simulink library "lib_Gimbal"  (R2017a)
settings: Solver=VariableStepAuto  StartTime=0.0  StopTime=10.0  RelTol=1e-3
undefined symbols (not defined in the file or in its folder): HIL_Data, HIL_Sample_Time, National_Instruments, PCIe, Standard_Devices, UDP_Protocol
libraries: sldrtlib x6, lib_Gimbal x5, sharedtransform x1
settings Model: Creator=m.hiepp  LastModifiedBy=m.hiepp
settings SFSimCC: SimUseLocalCustomCode=on
settings RTWCC: RTWUseLocalCustomCode=on

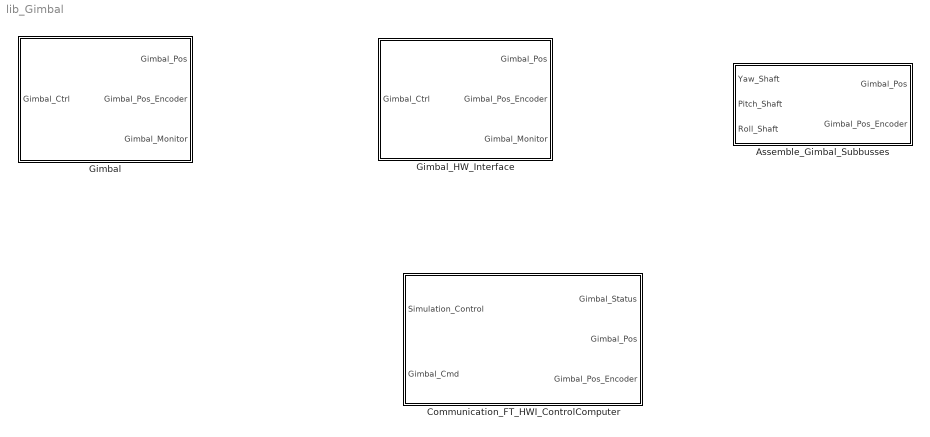
== system lib_Gimbal ==
  Assemble_Gimbal_Subbusses : Subsystem
  Communication_FT_HWI_ControlComputer : Subsystem  mask{FTHWICC=HIL_Data.Gimbal.FTHWICC}
      mask prompts: FTHWICC "FT HWI CC Connection Data"
  Gimbal : Subsystem  Variant=on
  Gimbal_HW_Interface : Subsystem  mask{HW=HIL_Data.Gimbal.HW}
      mask prompts: HW "HW Data"

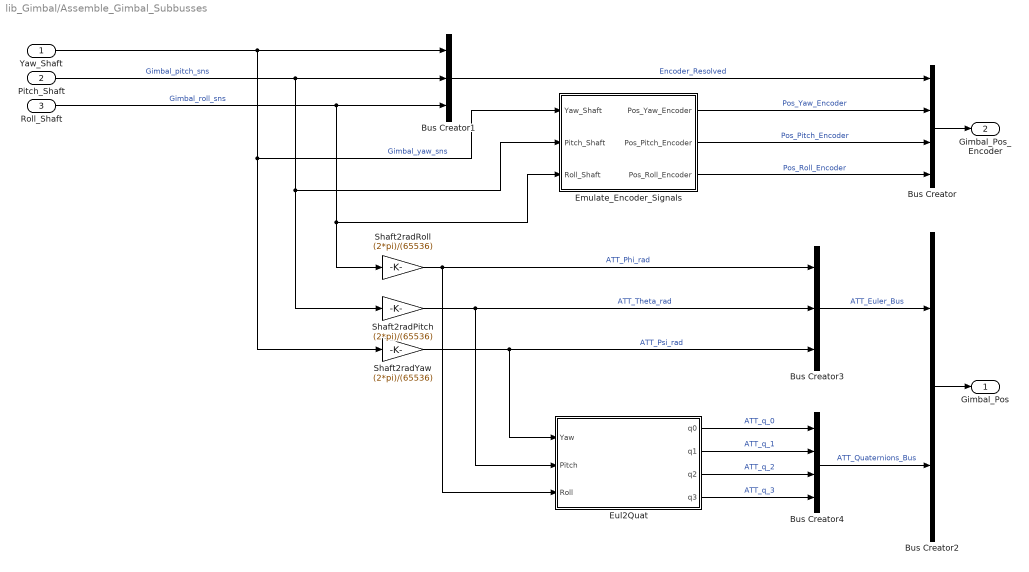
== system lib_Gimbal/Assemble_Gimbal_Subbusses ==
  Yaw_Shaft : Inport
  Pitch_Shaft : Inport  Port=2
  Roll_Shaft : Inport  Port=3
  Bus Creator : BusCreator  Inputs=4  OutDataTypeStr=Bus: Gimbal_Encoder_Bus
  Bus Creator1 : BusCreator  Inputs=3  OutDataTypeStr=Bus: Encoder_Resolved_Bus
  Bus Creator2 : BusCreator  Inputs=2  OutDataTypeStr=Bus: Attitude_States_Bus
  Bus Creator3 : BusCreator  Inputs=3  OutDataTypeStr=Bus: ATT_Euler_Bus
  Bus Creator4 : BusCreator  Inputs=4  OutDataTypeStr=Bus: ATT_Quaternions_Bus
  Emulate_Encoder_Signals : Subsystem
  Eul2Quat : Subsystem
  Shaft2radPitch : Gain  Gain=(2*pi)/(65536)
  Shaft2radRoll : Gain  Gain=(2*pi)/(65536)
  Shaft2radYaw : Gain  Gain=(2*pi)/(65536)
  Gimbal_Pos : Outport  OutDataTypeStr=Bus: Gimbal_Attitude_Bus
  Gimbal_Pos_Encoder : Outport  Port=2  OutDataTypeStr=Bus: Gimbal_Encoder_Bus
  wires:
  Roll_Shaft/1 -> Emulate_Encoder_Signals/3(Roll_Shaft), Shaft2radRoll/1, Bus Creator1/3  "Gimbal_roll_sns"
  Yaw_Shaft/1 -> Emulate_Encoder_Signals/1(Yaw_Shaft), Shaft2radYaw/1, Bus Creator1/1  "Gimbal_yaw_sns"
  Shaft2radPitch/1 -> Eul2Quat/2(Pitch), Bus Creator3/2  "ATT_Theta_rad"
  Bus Creator2/1 -> Gimbal_Pos/1
  Eul2Quat/4(q3) -> Bus Creator4/4  "ATT_q_3"
  Bus Creator/1 -> Gimbal_Pos_Encoder/1
  Eul2Quat/1(q0) -> Bus Creator4/1  "ATT_q_0"
  Pitch_Shaft/1 -> Emulate_Encoder_Signals/2(Pitch_Shaft), Shaft2radPitch/1, Bus Creator1/2  "Gimbal_pitch_sns"
  Eul2Quat/2(q1) -> Bus Creator4/2  "ATT_q_1"
  Bus Creator3/1 -> Bus Creator2/1  "ATT_Euler_Bus"
  Bus Creator4/1 -> Bus Creator2/2  "ATT_Quaternions_Bus"
  Bus Creator1/1 -> Bus Creator/1  "Encoder_Resolved"
  Shaft2radRoll/1 -> Eul2Quat/3(Roll), Bus Creator3/1  "ATT_Phi_rad"
  Shaft2radYaw/1 -> Eul2Quat/1(Yaw), Bus Creator3/3  "ATT_Psi_rad"
  Eul2Quat/3(q2) -> Bus Creator4/3  "ATT_q_2"
  Emulate_Encoder_Signals/1(Pos_Yaw_Encoder) -> Bus Creator/2  "Pos_Yaw_Encoder"
  Emulate_Encoder_Signals/2(Pos_Pitch_Encoder) -> Bus Creator/3  "Pos_Pitch_Encoder"
  Emulate_Encoder_Signals/3(Pos_Roll_Encoder) -> Bus Creator/4  "Pos_Roll_Encoder"

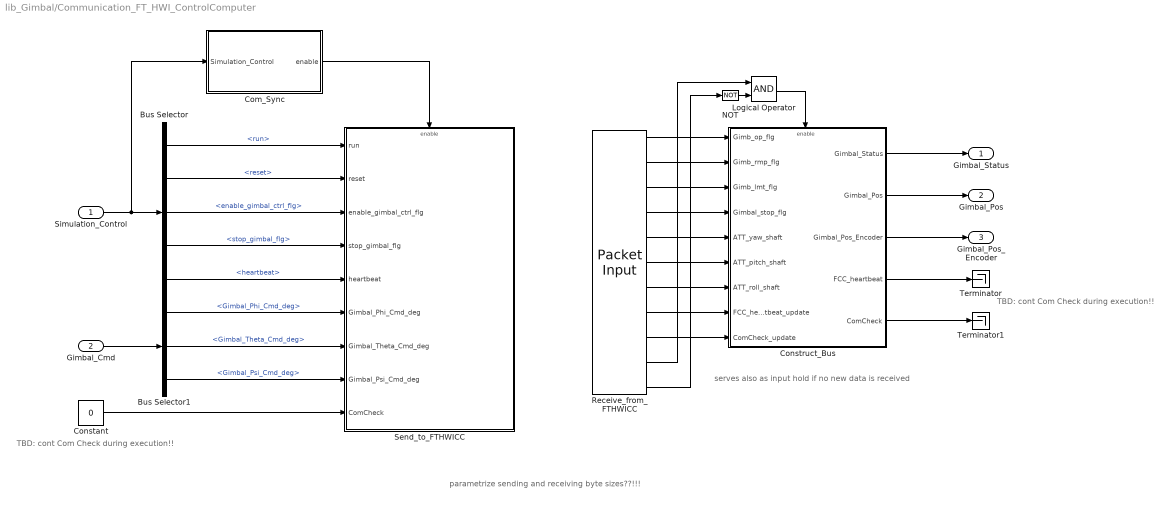
== system lib_Gimbal/Communication_FT_HWI_ControlComputer ==
  note: parametrize sending and receiving byte sizes??!!!
  note: TBD: cont Com Check during execution!!
  note: serves also as input hold if no new data is received
  note: TBD: cont Com Check during execution!!
  Simulation_Control : Inport  OutDataTypeStr=Bus: Simulation_Ctrl_Bus
  Gimbal_Cmd : Inport  Port=2  OutDataTypeStr=Bus: Gimbal_Cmd_Bus
  Bus Selector : BusSelector  OutputSignals=run,reset,HW_Ctrl.enable_gimbal_ctrl_flg,HW_Ctrl.stop_gimbal_flg,heartbeat
  Bus Selector1 : BusSelector  OutputSignals=Gimbal_Phi_Cmd_deg,Gimbal_Theta_Cmd_deg,Gimbal_Psi_Cmd_deg
  Com_Sync : Subsystem
  Constant : Constant  Value=0
  Construct_Bus : Subsystem
  Logical Operator : Logic  AllPortsSameDT=off  OutDataTypeStr=boolean
  NOT : Logic  Operator=NOT  IconShape=distinctive  AllPortsSameDT=off  OutDataTypeStr=boolean
  Receive_from_FTHWICC : sldrtlib/Packet Input  SampleTime=FTHWICC.SampTime  MaxMissedTicks=FTHWICC.MaxMissedTicks  ShowMissedTicks=off  YieldWhenWaiting=on  DrvName=Standard_Devices/UDP_Protocol  DrvAddress=36880  DrvOptions=[0 36864 0 0 0 0 0 0 0 0 0 0 0 0 0 0 0 0 0 0 0 0 0 0 0 0 0 0 0 0 0 0 0 0 0 0 0 0 0 0 0 0 0 0 0 0 0 0 0 0 0 0 0 0 0 0 0 0 0 0 0 0 0 0 0 0 0 0 0 0 0 0 0 0 0 0 0 0 0 0 0 0 0 0 0 0 0 0 0 0 0 0 0 0 0 0 0 0 0 0 0 0 0 0 0 0 0 0 0 0 0 0 0 0 0 0 0 0 0 0 0 0 0 0 0 0 0 0 0 0 0 0 0 0 0 0 0 0 0 0 0 0 0 0 0 0 0 0 0 0 0 0 0 0 0 0 0 0 0 0 0 0 0 0 0 0 0 0 0 0 0 0 0 0 0 0 0 0 0 0 0 0 0 0 0 0 0 0 0 0 0 0 0 0 0 0 0 0 0 0 0 0 0 0 0 0 0 0 0 0 0 0 0 0 0 0 0 0 0 0 0 0 0 0 0 0 0 0 0 0 0 0 0 0 0 0 0 0 0 0 0 0 0 0 0 0 0 0 0 0 0 0 0 0 0 0]  PacketSize=66  DataTypes={'double','double','double','double','double','double','double','uint16','double'}  ShowReady=on  ShowError=on  PacketID=1  ByteOrder=1  ShowTimestamp=off
      settings: AttributesFormatString=UDP Protocol [36880]  SourceProductName=Simulink Desktop Real-Time
  Send_to_FTHWICC : Subsystem
  Terminator : Terminator
  Terminator1 : Terminator
  Gimbal_Status : Outport  OutDataTypeStr=Bus: Gimbal_Status_Bus
  Gimbal_Pos : Outport  Port=2  OutDataTypeStr=Bus: Gimbal_Attitude_Bus
  Gimbal_Pos_Encoder : Outport  Port=3  OutDataTypeStr=Bus: Gimbal_Encoder_Bus
  wires:
  Simulation_Control/1 -> Com_Sync/1(Simulation_Control), Bus Selector/1
  Gimbal_Cmd/1 -> Bus Selector1/1
  Receive_from_FTHWICC/1 -> Construct_Bus/1(Gimb_op_flg)
  Receive_from_FTHWICC/2 -> Construct_Bus/2(Gimb_rmp_flg)
  Receive_from_FTHWICC/3 -> Construct_Bus/3(Gimb_lmt_flg)
  Receive_from_FTHWICC/4 -> Construct_Bus/4(Gimbal_stop_flg)
  Receive_from_FTHWICC/5 -> Construct_Bus/5(ATT_yaw_shaft)
  Receive_from_FTHWICC/6 -> Construct_Bus/6(ATT_pitch_shaft)
  Receive_from_FTHWICC/7 -> Construct_Bus/7(ATT_roll_shaft)
  Construct_Bus/1(Gimbal_Status) -> Gimbal_Status/1
  Construct_Bus/2(Gimbal_Pos) -> Gimbal_Pos/1
  Construct_Bus/3(Gimbal_Pos_Encoder) -> Gimbal_Pos_Encoder/1
  NOT/1 -> Logical Operator/2
  Receive_from_FTHWICC/10 -> Logical Operator/1
  Receive_from_FTHWICC/11 -> NOT/1
  Logical Operator/1 -> Construct_Bus/Enable
  Bus Selector/1 -> Send_to_FTHWICC/1(run)  "<run>"
  Bus Selector/2 -> Send_to_FTHWICC/2(reset)  "<reset>"
  Bus Selector/3 -> Send_to_FTHWICC/3(enable_gimbal_ctrl_flg)  "<enable_gimbal_ctrl_flg>"
  Bus Selector/4 -> Send_to_FTHWICC/4(stop_gimbal_flg)  "<stop_gimbal_flg>"
  Bus Selector/5 -> Send_to_FTHWICC/5(heartbeat)  "<heartbeat>"
  Bus Selector1/1 -> Send_to_FTHWICC/6(Gimbal_Phi_Cmd_deg)  "<Gimbal_Phi_Cmd_deg>"
  Bus Selector1/2 -> Send_to_FTHWICC/7(Gimbal_Theta_Cmd_deg)  "<Gimbal_Theta_Cmd_deg>"
  Bus Selector1/3 -> Send_to_FTHWICC/8(Gimbal_Psi_Cmd_deg)  "<Gimbal_Psi_Cmd_deg>"
  Com_Sync/1(enable) -> Send_to_FTHWICC/Enable
  Constant/1 -> Send_to_FTHWICC/9(ComCheck)
  Receive_from_FTHWICC/8 -> Construct_Bus/8(FCC_heartbeat_update)
  Receive_from_FTHWICC/9 -> Construct_Bus/9(ComCheck_update)
  Construct_Bus/4(FCC_heartbeat) -> Terminator/1
  Construct_Bus/5(ComCheck) -> Terminator1/1

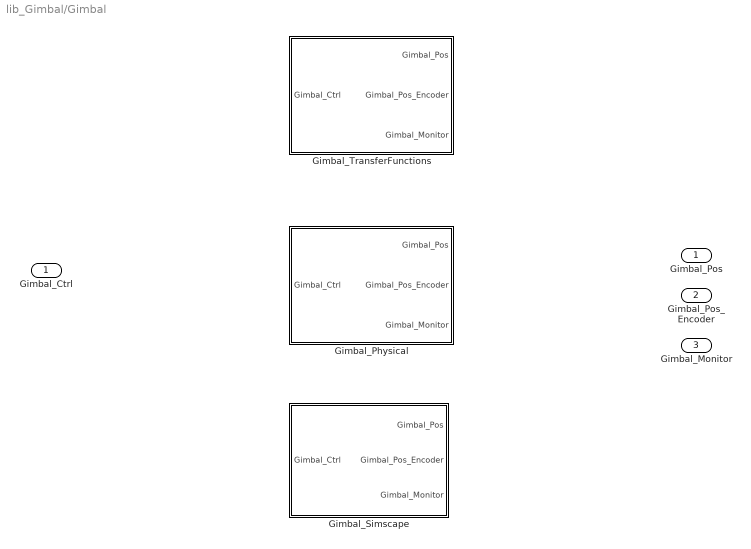
== system lib_Gimbal/Gimbal ==
  Gimbal_Ctrl : Inport  OutDataTypeStr=Bus: Gimbal_Ctrl_Bus
  Gimbal_Physical : Subsystem  VariantControl=VSS_GIMBAL_PH
  Gimbal_Simscape : Subsystem  VariantControl=VSS_GIMBAL_SC
  Gimbal_TransferFunctions : Subsystem  VariantControl=VSS_GIMBAL_TF  mask{TF=HIL_Data.Gimbal.TF}
      mask prompts: TF "Transfer_Functions"
  Gimbal_Pos : Outport  OutDataTypeStr=Bus: Gimbal_Attitude_Bus
  Gimbal_Pos_Encoder : Outport  Port=2  OutDataTypeStr=Bus: Gimbal_Encoder_Bus
  Gimbal_Monitor : Outport  Port=3  OutDataTypeStr=Bus: Gimbal_Monitor_Bus

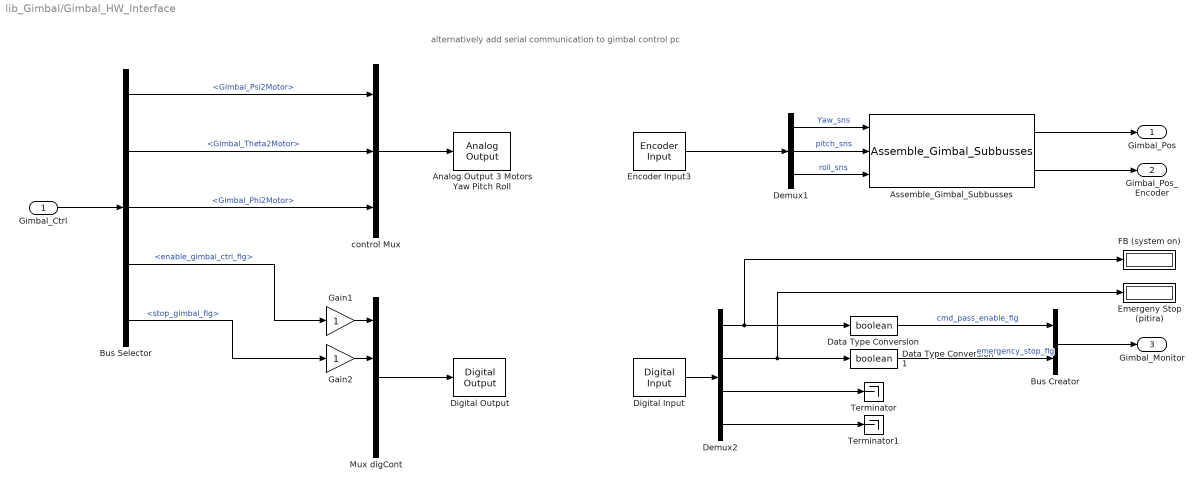
== system lib_Gimbal/Gimbal_HW_Interface ==
  note: alternatively add serial communication to gimbal control pc
  Gimbal_Ctrl : Inport  OutDataTypeStr=Bus: Gimbal_Ctrl_Bus
  Analog Output 3 Motors Yaw Pitch Roll : sldrtlib/Analog Output  SampleTime=HW.SampTime  MaxMissedTicks=HW.MaxMissTick  ShowMissedTicks=off  YieldWhenWaiting=off  DrvName=National_Instruments/PCIe-6353  DrvAddress=4294967295  DrvOptions=[0 15 0 2 2 2 2]  Channels=[1:3]  RangeMode=1  VoltRange=1  InitialValue=0  FinalValue=0
      settings: AttributesFormatString=National Instruments\nPCIe-6353 [auto]  SourceProductName=Simulink Desktop Real-Time
  Assemble_Gimbal_Subbusses : lib_Gimbal/Assemble_Gimbal_Subbusses  SystemSampleTime=-1
  Bus Creator : BusCreator  Inputs=2  OutDataTypeStr=Bus: Gimbal_Monitor_Bus
  Bus Selector : BusSelector  OutputSignals=Gimbal_Psi2Motor,Gimbal_Theta2Motor,Gimbal_Phi2Motor,enable_gimbal_ctrl_flg,stop_gimbal_flg
  Data Type Conversion : DataTypeConversion  OutDataTypeStr=boolean
  Data Type Conversion1 : DataTypeConversion  OutDataTypeStr=boolean
  Demux1 : Demux  Outputs=3
  Demux2 : Demux
  Digital Input : sldrtlib/Digital Input  SampleTime=HW.SampTime  MaxMissedTicks=HW.MaxMissTick  ShowMissedTicks=off  YieldWhenWaiting=off  DrvName=National_Instruments/PCIe-6353  DrvAddress=4294967295  DrvOptions=[0 15 0 2 2 2 2]  Channels=[5:8]  BitMode=1  DataType=1
      settings: AttributesFormatString=National Instruments\nPCIe-6353 [auto]  SourceProductName=Simulink Desktop Real-Time  SourceProductBaseCode=WT
  Digital Output : sldrtlib/Digital Output  SampleTime=HW.SampTime  MaxMissedTicks=HW.MaxMissTick  ShowMissedTicks=off  YieldWhenWaiting=off  DrvName=National_Instruments/PCIe-6353  DrvAddress=4294967295  DrvOptions=[0 15 0 2 2 2 2]  Channels=[1:4]  BitMode=1  InitialValue=[]  FinalValue=[]
      settings: AttributesFormatString=National Instruments\nPCIe-6353 [auto]  SourceProductName=Simulink Desktop Real-Time  SourceProductBaseCode=WT
  Emergeny Stop (pitira) : Display
      settings: Tag=SampTime
  Encoder Input3 : sldrtlib/Encoder Input  SampleTime=HW.SampTime  MaxMissedTicks=HW.MaxMissTick  ShowMissedTicks=off  YieldWhenWaiting=off  DrvName=National_Instruments/PCIe-6353  DrvAddress=4294967295  DrvOptions=[0 15 0 2 2 2 2]  Channels=[1:3]  QuadMode=3  IndexPulse=1  InputFilter=Inf  DataType=1
      settings: AttributesFormatString=National Instruments\nPCIe-6353 [auto]  SourceProductName=Simulink Desktop Real-Time
  FB (system on) : Display
      settings: Tag=SampTime
  Gain1 : Gain
  Gain2 : Gain
  Mux digCont : Mux
  Terminator : Terminator
  Terminator1 : Terminator
  control Mux : Mux  Inputs=3
  Gimbal_Pos : Outport  OutDataTypeStr=Bus: Gimbal_Attitude_Bus
  Gimbal_Pos_Encoder : Outport  Port=2  OutDataTypeStr=Bus: Gimbal_Encoder_Bus
  Gimbal_Monitor : Outport  Port=3  OutDataTypeStr=Bus: Gimbal_Monitor_Bus
  wires:
  Assemble_Gimbal_Subbusses/2 -> Gimbal_Pos_Encoder/1
  Gimbal_Ctrl/1 -> Bus Selector/1
  Assemble_Gimbal_Subbusses/1 -> Gimbal_Pos/1
  control Mux/1 -> Analog Output 3 Motors Yaw Pitch Roll/1
  Demux1/3 -> Assemble_Gimbal_Subbusses/3  "roll_sns"
  Demux1/1 -> Assemble_Gimbal_Subbusses/1  "Yaw_sns"
  Demux1/2 -> Assemble_Gimbal_Subbusses/2  "pitch_sns"
  Encoder Input3/1 -> Demux1/1
  Bus Selector/1 -> control Mux/1  "<Gimbal_Psi2Motor>"
  Bus Selector/2 -> control Mux/2  "<Gimbal_Theta2Motor>"
  Bus Selector/3 -> control Mux/3  "<Gimbal_Phi2Motor>"
  Demux2/1 -> Data Type Conversion/1, FB (system on)/1
  Digital Input/1 -> Demux2/1
  Mux digCont/1 -> Digital Output/1
  Demux2/2 -> Data Type Conversion1/1, Emergeny Stop (pitira)/1
  Bus Creator/1 -> Gimbal_Monitor/1
  Data Type Conversion/1 -> Bus Creator/1  "cmd_pass_enable_flg"
  Data Type Conversion1/1 -> Bus Creator/2  "emergency_stop_flg"
  Demux2/3 -> Terminator/1
  Demux2/4 -> Terminator1/1
  Bus Selector/4 -> Gain1/1  "<enable_gimbal_ctrl_flg>"
  Gain1/1 -> Mux digCont/1
  Gain2/1 -> Mux digCont/2
  Bus Selector/5 -> Gain2/1  "<stop_gimbal_flg>"

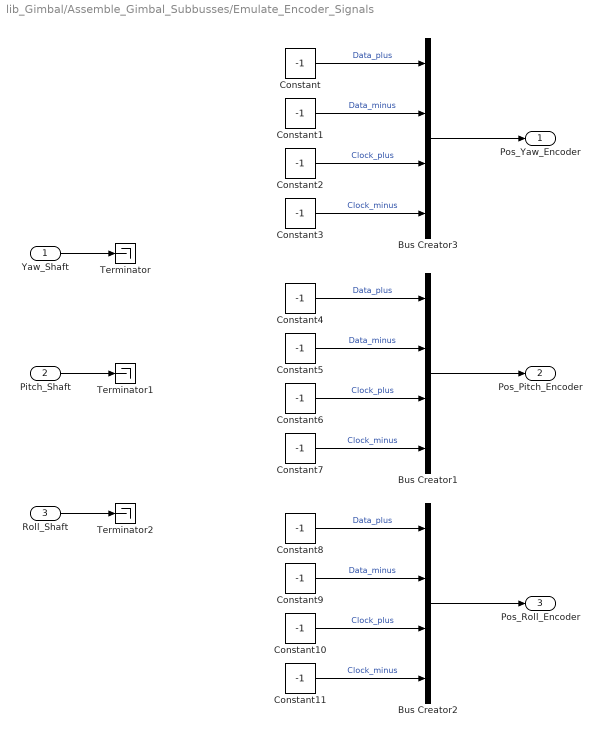
== system lib_Gimbal/Assemble_Gimbal_Subbusses/Emulate_Encoder_Signals ==
  Yaw_Shaft : Inport
  Pitch_Shaft : Inport  Port=2
  Roll_Shaft : Inport  Port=3
  Bus Creator1 : BusCreator  Inputs=4  OutDataTypeStr=Bus: Encoder_Signal_Bus
  Bus Creator2 : BusCreator  Inputs=4  OutDataTypeStr=Bus: Encoder_Signal_Bus
  Bus Creator3 : BusCreator  Inputs=4  OutDataTypeStr=Bus: Encoder_Signal_Bus
  Constant{,1..11} (12 alike) : Constant  Value=-1
  Terminator : Terminator
  Terminator1 : Terminator
  Terminator2 : Terminator
  Pos_Yaw_Encoder : Outport  OutDataTypeStr=Bus: Encoder_Signal_Bus
  Pos_Pitch_Encoder : Outport  Port=2  OutDataTypeStr=Bus: Encoder_Signal_Bus
  Pos_Roll_Encoder : Outport  Port=3  OutDataTypeStr=Bus: Encoder_Signal_Bus
  wires:
  Bus Creator2/1 -> Pos_Roll_Encoder/1
  Yaw_Shaft/1 -> Terminator/1
  Pitch_Shaft/1 -> Terminator1/1
  Roll_Shaft/1 -> Terminator2/1
  Bus Creator3/1 -> Pos_Yaw_Encoder/1
  Bus Creator1/1 -> Pos_Pitch_Encoder/1
  Constant/1 -> Bus Creator3/1  "Data_plus"
  Constant11/1 -> Bus Creator2/4  "Clock_minus"
  Constant10/1 -> Bus Creator2/3  "Clock_plus"
  Constant9/1 -> Bus Creator2/2  "Data_minus"
  Constant8/1 -> Bus Creator2/1  "Data_plus"
  Constant7/1 -> Bus Creator1/4  "Clock_minus"
  Constant6/1 -> Bus Creator1/3  "Clock_plus"
  Constant5/1 -> Bus Creator1/2  "Data_minus"
  Constant3/1 -> Bus Creator3/4  "Clock_minus"
  Constant4/1 -> Bus Creator1/1  "Data_plus"
  Constant2/1 -> Bus Creator3/3  "Clock_plus"
  Constant1/1 -> Bus Creator3/2  "Data_minus"

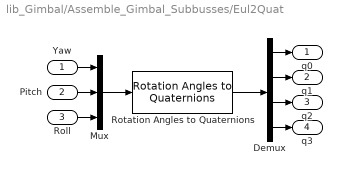
== system lib_Gimbal/Assemble_Gimbal_Subbusses/Eul2Quat ==
  Yaw : Inport
  Pitch : Inport  Port=2
  Roll : Inport  Port=3
  Demux : Demux
  Mux : Mux  Inputs=3
  Rotation Angles to Quaternions : sharedtransform/Rotation Angles to Quaternions  rotationOrder=XYZ
      settings: SourceProductName=Aerospace Blockset  SourceProductBaseCode=AE
  q0 : Outport
  q1 : Outport  Port=2
  q2 : Outport  Port=3
  q3 : Outport  Port=4
  wires:
  Demux/2 -> q1/1
  Pitch/1 -> Mux/2
  Rotation Angles to Quaternions/1 -> Demux/1
  Mux/1 -> Rotation Angles to Quaternions/1
  Demux/4 -> q3/1
  Roll/1 -> Mux/3
  Demux/3 -> q2/1
  Yaw/1 -> Mux/1
  Demux/1 -> q0/1

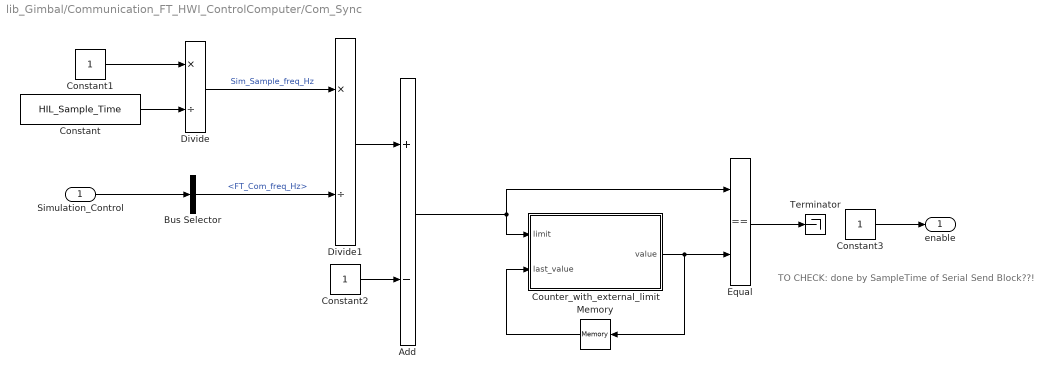
== system lib_Gimbal/Communication_FT_HWI_ControlComputer/Com_Sync ==
  note: TO CHECK: done by SampleTime of Serial Send Block??!
  Simulation_Control : Inport  OutDataTypeStr=Bus: Simulation_Ctrl_Bus
  Add : Sum  Inputs=+-
  Bus Selector : BusSelector  OutputSignals=COM_Ctrl.FT_Com_freq_Hz
  Constant : Constant  Value=HIL_Sample_Time
  Constant1 : Constant
  Constant2 : Constant
  Constant3 : Constant  OutDataTypeStr=boolean
  Counter_with_external_limit : MATLAB Function  TreatAsAtomicUnit=on
  Divide : Product  Inputs=*/
  Divide1 : Product  Inputs=*/
  Equal : RelationalOperator  Operator===  OutDataTypeStr=boolean  RndMeth=Simplest
  Memory : Memory  X0=-1
  Terminator : Terminator
  enable : Outport
  wires:
  Simulation_Control/1 -> Bus Selector/1
  Constant/1 -> Divide/2
  Constant1/1 -> Divide/1
  Divide/1 -> Divide1/1  "Sim_Sample_freq_Hz"
  Bus Selector/1 -> Divide1/2  "<FT_Com_freq_Hz>"
  Divide1/1 -> Add/1
  Constant2/1 -> Add/2
  Counter_with_external_limit/1(value) -> Memory/1, Equal/2
  Memory/1 -> Counter_with_external_limit/2(last_value)
  Add/1 -> Equal/1, Counter_with_external_limit/1(limit)
  Equal/1 -> Terminator/1
  Constant3/1 -> enable/1

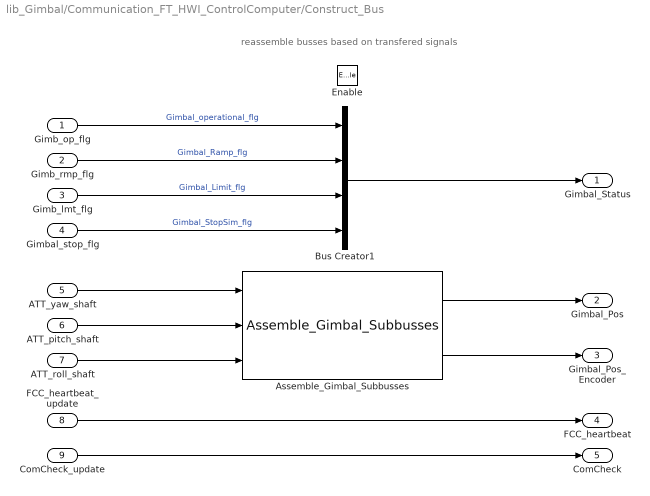
== system lib_Gimbal/Communication_FT_HWI_ControlComputer/Construct_Bus ==
  note: reassemble busses based on transfered signals
  Gimb_op_flg : Inport
  Gimb_rmp_flg : Inport  Port=2
  Gimb_lmt_flg : Inport  Port=3
  Gimbal_stop_flg : Inport  Port=4
  ATT_yaw_shaft : Inport  Port=5
  ATT_pitch_shaft : Inport  Port=6
  ATT_roll_shaft : Inport  Port=7
  FCC_heartbeat_update : Inport  Port=8
  ComCheck_update : Inport  Port=9
  Enable : EnablePort
  Assemble_Gimbal_Subbusses : lib_Gimbal/Assemble_Gimbal_Subbusses  SystemSampleTime=-1
  Bus Creator1 : BusCreator  Inputs=4
  Gimbal_Status : Outport  OutDataTypeStr=Bus: Gimbal_Status_Bus
  Gimbal_Pos : Outport  Port=2  OutDataTypeStr=Bus: Gimbal_Attitude_Bus
  Gimbal_Pos_Encoder : Outport  Port=3  OutDataTypeStr=Bus: Gimbal_Encoder_Bus
  FCC_heartbeat : Outport  Port=4
  ComCheck : Outport  Port=5
  wires:
  Gimb_lmt_flg/1 -> Bus Creator1/3  "Gimbal_Limit_flg"
  Gimbal_stop_flg/1 -> Bus Creator1/4  "Gimbal_StopSim_flg"
  Gimb_rmp_flg/1 -> Bus Creator1/2  "Gimbal_Ramp_flg"
  Gimb_op_flg/1 -> Bus Creator1/1  "Gimbal_operational_flg"
  Bus Creator1/1 -> Gimbal_Status/1
  ATT_yaw_shaft/1 -> Assemble_Gimbal_Subbusses/1
  ATT_pitch_shaft/1 -> Assemble_Gimbal_Subbusses/2
  ATT_roll_shaft/1 -> Assemble_Gimbal_Subbusses/3
  Assemble_Gimbal_Subbusses/1 -> Gimbal_Pos/1
  Assemble_Gimbal_Subbusses/2 -> Gimbal_Pos_Encoder/1
  FCC_heartbeat_update/1 -> FCC_heartbeat/1
  ComCheck_update/1 -> ComCheck/1

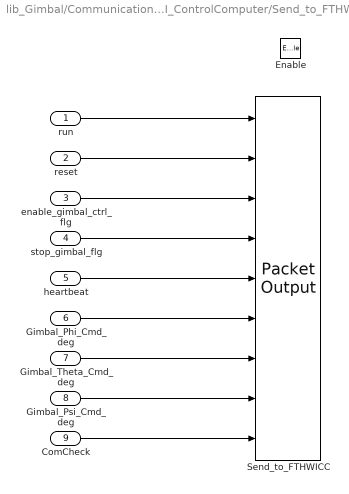
== system lib_Gimbal/Communication_FT_HWI_ControlComputer/Send_to_FTHWICC ==
  run : Inport
  reset : Inport  Port=2
  enable_gimbal_ctrl_flg : Inport  Port=3
  stop_gimbal_flg : Inport  Port=4
  heartbeat : Inport  Port=5
  Gimbal_Phi_Cmd_deg : Inport  Port=6
  Gimbal_Theta_Cmd_deg : Inport  Port=7
  Gimbal_Psi_Cmd_deg : Inport  Port=8
  ComCheck : Inport  Port=9
  Enable : EnablePort
  Send_to_FTHWICC : sldrtlib/Packet Output  SampleTime=1/HIL_Data.Simulation_Ctrl.Com.FT.Com_freq_Hz  MaxMissedTicks=FTHWICC.MaxMissTick  ShowMissedTicks=off  YieldWhenWaiting=on  DrvName=Standard_Devices/UDP_Protocol  DrvAddress=36864  DrvOptions=[0 36880 49 57 50 46 49 54 56 46 49 46 49 53 54 0 0 0 0 0 0 0 0 0 0 0 0 0 0 0 0 0 0 0 0 0 0 0 0 0 0 0 0 0 0 0 0 0 0 0 0 0 0 0 0 0 0 0 0 0 0 0 0 0 0 0 0 0 0 0 0 0 0 0 0 0 0 0 0 0 0 0 0 0 0 0 0 0 0 0 0 0 0 0 0 0 0 0 0 0 0 0 0 0 0 0 0 0 0 0 0 0 0 0 0 0 0 0 0 0 0 0 0 0 0 0 0 0 0 0 0 0 0 0 0 0 0 0 0 0 0 0 0 0 0 0 0 0 0 0 0 0 0 0 0 0 0 0 0 0 0 0 0 0 0 0 0 0 0 0 0 0 0 0 0 0 0 0 0 0 0 0 0 0 0 0 0 0 0 0 0 0 0 0 0 0 0 0 0 0 0 0 0 0 0 0 0 0 0 0 0 0 0 0 0 0 0 0 0 0 0 0 0 0 0 0 0 0 0 0 0 0 0 0 0 0 0 0 0 0 0 0 0 0 0 0 0 0 0 0 0 0 0 0 0 0]  PacketSize=52  DataTypes={'boolean','boolean','double','double','uint16','double','double','double','double'}  ShowReady=off  ShowError=off  PacketID=1  ByteOrder=1  InitialValue=[]  FinalValue=[]
      settings: AttributesFormatString=UDP Protocol [36864]  SourceProductName=Simulink Desktop Real-Time
  wires:
  Gimbal_Psi_Cmd_deg/1 -> Send_to_FTHWICC/8
  heartbeat/1 -> Send_to_FTHWICC/5
  Gimbal_Theta_Cmd_deg/1 -> Send_to_FTHWICC/7
  reset/1 -> Send_to_FTHWICC/2
  Gimbal_Phi_Cmd_deg/1 -> Send_to_FTHWICC/6
  stop_gimbal_flg/1 -> Send_to_FTHWICC/4
  run/1 -> Send_to_FTHWICC/1
  enable_gimbal_ctrl_flg/1 -> Send_to_FTHWICC/3
  ComCheck/1 -> Send_to_FTHWICC/9

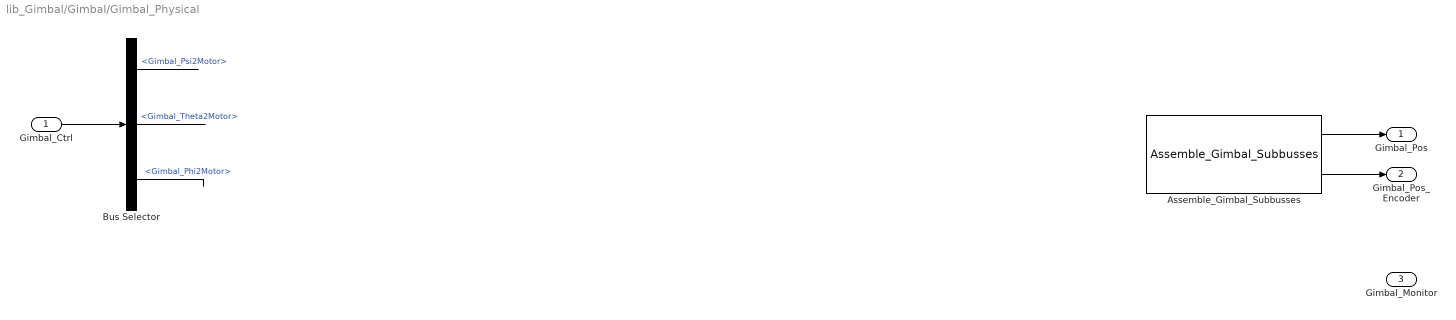
== system lib_Gimbal/Gimbal/Gimbal_Physical ==
  Gimbal_Ctrl : Inport  OutDataTypeStr=Bus: Gimbal_Ctrl_Bus
  Assemble_Gimbal_Subbusses : lib_Gimbal/Assemble_Gimbal_Subbusses  SystemSampleTime=-1
  Bus Selector : BusSelector  OutputSignals=Gimbal_Psi2Motor,Gimbal_Theta2Motor,Gimbal_Phi2Motor
  Gimbal_Pos : Outport  OutDataTypeStr=Bus: Gimbal_Attitude_Bus
  Gimbal_Pos_Encoder : Outport  Port=2  OutDataTypeStr=Bus: Gimbal_Encoder_Bus
  Gimbal_Monitor : Outport  Port=3  OutDataTypeStr=Bus: Gimbal_Monitor_Bus
  wires:
  Gimbal_Ctrl/1 -> Bus Selector/1
  Assemble_Gimbal_Subbusses/1 -> Gimbal_Pos/1
  Assemble_Gimbal_Subbusses/2 -> Gimbal_Pos_Encoder/1
  Bus Selector/1 -> ?  "<Gimbal_Psi2Motor>"
  Bus Selector/2 -> ?  "<Gimbal_Theta2Motor>"
  Bus Selector/3 -> ?  "<Gimbal_Phi2Motor>"

== system lib_Gimbal/Gimbal/Gimbal_Simscape ==
  Gimbal_Ctrl : Inport  OutDataTypeStr=Bus: Gimbal_Ctrl_Bus
  Assemble_Gimbal_Subbusses : lib_Gimbal/Assemble_Gimbal_Subbusses  SystemSampleTime=-1
  Bus Selector : BusSelector  OutputSignals=Gimbal_Psi2Motor,Gimbal_Theta2Motor,Gimbal_Phi2Motor
  Gimbal_Pos : Outport  OutDataTypeStr=Bus: Gimbal_Attitude_Bus
  Gimbal_Pos_Encoder : Outport  Port=2  OutDataTypeStr=Bus: Gimbal_Encoder_Bus
  Gimbal_Monitor : Outport  Port=3  OutDataTypeStr=Bus: Gimbal_Monitor_Bus
  wires:
  Bus Selector/3 -> ?  "<Gimbal_Phi2Motor>"
  Gimbal_Ctrl/1 -> Bus Selector/1
  Bus Selector/2 -> ?  "<Gimbal_Theta2Motor>"
  Assemble_Gimbal_Subbusses/1 -> Gimbal_Pos/1
  Assemble_Gimbal_Subbusses/2 -> Gimbal_Pos_Encoder/1
  Bus Selector/1 -> ?  "<Gimbal_Psi2Motor>"

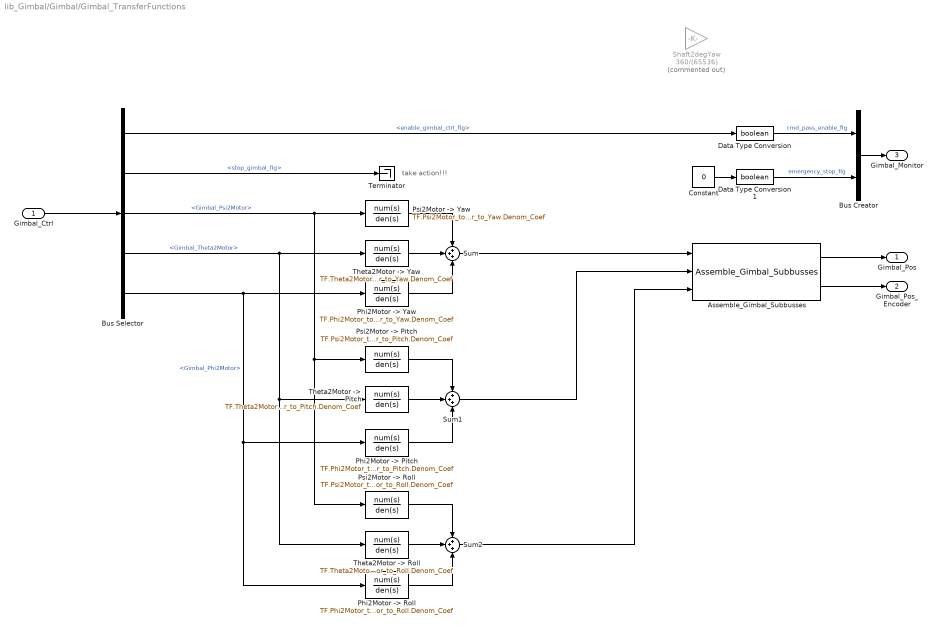
== system lib_Gimbal/Gimbal/Gimbal_TransferFunctions ==
  note: take action!!!
  Gimbal_Ctrl : Inport  OutDataTypeStr=Bus: Gimbal_Ctrl_Bus
  Assemble_Gimbal_Subbusses : lib_Gimbal/Assemble_Gimbal_Subbusses  SystemSampleTime=-1
  Bus Creator : BusCreator  Inputs=2  OutDataTypeStr=Bus: Gimbal_Monitor_Bus
  Bus Selector : BusSelector  OutputSignals=enable_gimbal_ctrl_flg,stop_gimbal_flg,Gimbal_Psi2Motor,Gimbal_Theta2Motor,Gimbal_Phi2Motor
  Constant : Constant  Value=0
  Data Type Conversion : DataTypeConversion  OutDataTypeStr=boolean
  Data Type Conversion1 : DataTypeConversion  OutDataTypeStr=boolean
  "Phi2Motor -> Pitch" : TransferFcn  Numerator=TF.Phi2Motor_to_Pitch.Num_Coef  Denominator=TF.Phi2Motor_to_Pitch.Denom_Coef
  "Phi2Motor -> Roll" : TransferFcn  Numerator=TF.Phi2Motor_to_Roll.Num_Coef  Denominator=TF.Phi2Motor_to_Roll.Denom_Coef
  "Phi2Motor -> Yaw" : TransferFcn  Numerator=TF.Phi2Motor_to_Yaw.Num_Coef  Denominator=TF.Phi2Motor_to_Yaw.Denom_Coef
  "Psi2Motor -> Pitch" : TransferFcn  Numerator=TF.Psi2Motor_to_Pitch.Num_Coef  Denominator=TF.Psi2Motor_to_Pitch.Denom_Coef
  "Psi2Motor -> Roll" : TransferFcn  Numerator=TF.Psi2Motor_to_Roll.Num_Coef  Denominator=TF.Psi2Motor_to_Roll.Denom_Coef
  "Psi2Motor -> Yaw" : TransferFcn  Numerator=TF.Psi2Motor_to_Yaw.Num_Coef  Denominator=TF.Psi2Motor_to_Yaw.Denom_Coef
  Shaft2degYaw : Gain  Commented=on  Gain=360/(65536)
  Sum : Sum  Inputs=+++
  Sum1 : Sum  Inputs=+++
  Sum2 : Sum  Inputs=+++
  Terminator : Terminator
  "Theta2Motor -> Pitch" : TransferFcn  Numerator=TF.Theta2Motor_to_Pitch.Num_Coef  Denominator=TF.Theta2Motor_to_Pitch.Denom_Coef
  "Theta2Motor -> Roll" : TransferFcn  Numerator=TF.Theta2Motor_to_Roll.Num_Coef  Denominator=TF.Theta2Motor_to_Roll.Denom_Coef
  "Theta2Motor -> Yaw" : TransferFcn  Numerator=TF.Theta2Motor_to_Yaw.Num_Coef  Denominator=TF.Theta2Motor_to_Yaw.Denom_Coef
  Gimbal_Pos : Outport  OutDataTypeStr=Bus: Gimbal_Attitude_Bus
  Gimbal_Pos_Encoder : Outport  Port=2  OutDataTypeStr=Bus: Gimbal_Encoder_Bus
  Gimbal_Monitor : Outport  Port=3  OutDataTypeStr=Bus: Gimbal_Monitor_Bus
  wires:
  Gimbal_Ctrl/1 -> Bus Selector/1
  Bus Selector/5 -> "Phi2Motor -> Yaw"/1, "Phi2Motor -> Pitch"/1, "Phi2Motor -> Roll"/1  "<Gimbal_Phi2Motor>"
  Bus Selector/4 -> "Theta2Motor -> Yaw"/1, "Theta2Motor -> Pitch"/1, "Theta2Motor -> Roll"/1  "<Gimbal_Theta2Motor>"
  Bus Selector/3 -> "Psi2Motor -> Yaw"/1, "Psi2Motor -> Pitch"/1, "Psi2Motor -> Roll"/1  "<Gimbal_Psi2Motor>"
  "Theta2Motor -> Roll"/1 -> Sum2/2
  "Theta2Motor -> Pitch"/1 -> Sum1/2
  "Theta2Motor -> Yaw"/1 -> Sum/2
  "Psi2Motor -> Yaw"/1 -> Sum/1
  "Phi2Motor -> Yaw"/1 -> Sum/3
  "Psi2Motor -> Pitch"/1 -> Sum1/1
  "Phi2Motor -> Pitch"/1 -> Sum1/3
  "Psi2Motor -> Roll"/1 -> Sum2/1
  "Phi2Motor -> Roll"/1 -> Sum2/3
  Sum/1 -> Assemble_Gimbal_Subbusses/1
  Sum1/1 -> Assemble_Gimbal_Subbusses/2
  Sum2/1 -> Assemble_Gimbal_Subbusses/3
  Assemble_Gimbal_Subbusses/1 -> Gimbal_Pos/1
  Assemble_Gimbal_Subbusses/2 -> Gimbal_Pos_Encoder/1
  Bus Creator/1 -> Gimbal_Monitor/1
  Bus Selector/1 -> Data Type Conversion/1  "<enable_gimbal_ctrl_flg>"
  Bus Selector/2 -> Terminator/1  "<stop_gimbal_flg>"
  Constant/1 -> Data Type Conversion1/1
  Data Type Conversion/1 -> Bus Creator/1  "cmd_pass_enable_flg"
  Data Type Conversion1/1 -> Bus Creator/2  "emergency_stop_flg"

== matlab function lib_Gimbal/Communication_FT_HWI_ControlComputer/Com_Sync/Counter_with_external_limit ==
  data: limit input; value output; last_value input
function value = Counter(limit,last_value)
    
    if last_value < limit
        value = last_value + 1;
    else
        value = 0;
    end
    
end
